simulink subsystem "LQR"  (R2024a)
settings: Solver=VariableStepAuto  StartTime=0.0  StopTime=10.0  RelTol=1e-3
undefined symbols (not defined in the file): LQR, u_eq, x_eq
settings Model: Creator=Bocchio  LastModifiedBy=Bocchio

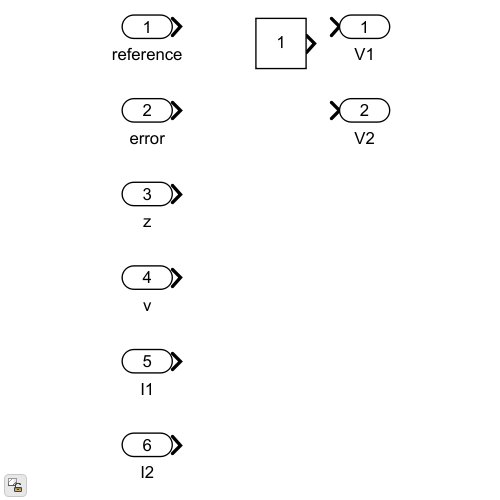
[thumbnail: Simulink's stored preview of the top-level diagram]
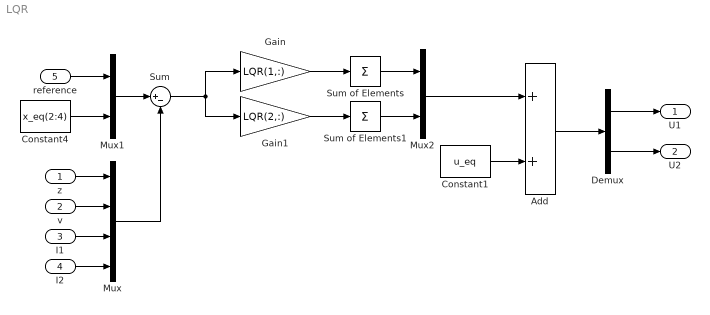
== system LQR ==
  z : Inport
  v : Inport  Port=2
  I1 : Inport  Port=3
  I2 : Inport  Port=4
  reference : Inport  Port=5
  Add : Sum
  Constant1 : Constant  Value=u_eq
  Constant4 : Constant  Value=x_eq(2:4)
  Demux : Demux  Outputs=2
  Gain : Gain  Gain=LQR(1,:)
  Gain1 : Gain  Gain=LQR(2,:)
  Mux : Mux
  Mux1 : Mux  Inputs=2
  Mux2 : Mux  Inputs=2
  Sum : Sum  Inputs=|+-
  Sum of Elements : Sum  Inputs=+  CollapseDim=2
  Sum of Elements1 : Sum  Inputs=+  CollapseDim=2
  U1 : Outport
  U2 : Outport  Port=2
  wires:
  Demux/2 -> U2/1
  Gain/1 -> Sum of Elements/1
  Add/1 -> Demux/1
  Constant1/1 -> Add/2
  Constant4/1 -> Mux1/2
  z/1 -> Mux/1
  v/1 -> Mux/2
  I1/1 -> Mux/3
  I2/1 -> Mux/4
  reference/1 -> Mux1/1
  Mux1/1 -> Sum/1
  Mux/1 -> Sum/2
  Mux2/1 -> Add/1
  Demux/1 -> U1/1
  Gain1/1 -> Sum of Elements1/1
  Sum/1 -> Gain/1, Gain1/1
  Sum of Elements/1 -> Mux2/1
  Sum of Elements1/1 -> Mux2/2
